simulink model "simlinkdatei_angelos_aufgabe"  (Simulink 7.9)
settings: Solver=ode45  StartTime=0.0  StopTime=10.0  RelTol=1e-3
settings Model: Creator=s67750  LastModifiedBy=s67750

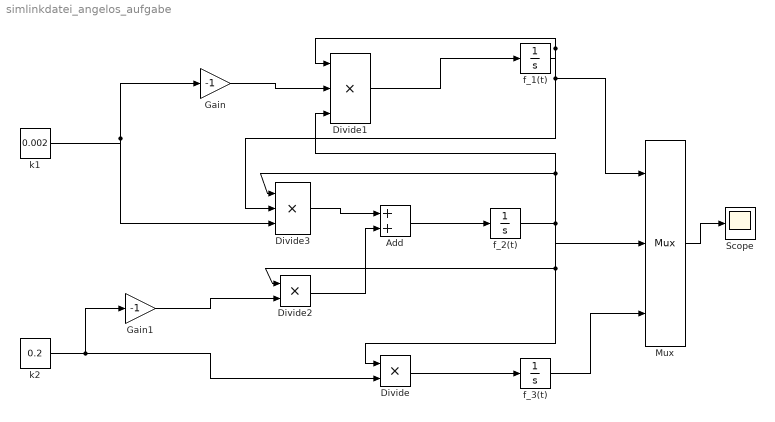
== system simlinkdatei_angelos_aufgabe ==
  Add : Sum
  Divide : Product  Inputs=**
  Divide1 : Product  Inputs=***
  Divide2 : Product  Inputs=**
  Divide3 : Product  Inputs=***
  Gain : Gain  Gain=-1
  Gain1 : Gain  Gain=-1
  Mux : Mux  Inputs=3
      settings: DisplayOption=signals
  Scope : Scope
  f_1(t) : Integrator  InitialCondition=1000
  f_2(t) : Integrator  InitialCondition=500
  f_3(t) : Integrator  InitialCondition=200
  k1 : Constant  Value=0.002
  k2 : Constant  Value=0.2
  wires:
  Divide/1 -> f_3(t)/1
  f_2(t)/1 -> Divide/1, Divide2/1, Divide1/3, Divide3/1, Mux/2
  k2/1 -> Divide/2, Gain1/1
  k1/1 -> Gain/1, Divide3/3
  f_1(t)/1 -> Divide1/1, Divide3/2, Mux/1
  Gain/1 -> Divide1/2
  Divide1/1 -> f_1(t)/1
  Gain1/1 -> Divide2/2
  Add/1 -> f_2(t)/1
  Divide2/1 -> Add/2
  Divide3/1 -> Add/1
  Mux/1 -> Scope/1
  f_3(t)/1 -> Mux/3
